simulink model "Controlador_PD"  (R2023a)
settings: Solver=ode1  StartTime=0.0  StopTime=10.0  FixedStep=0.01  RelTol=1e-3
settings Model: Creator=Nacho Andrade  LastModifiedBy=Nacho Andrade

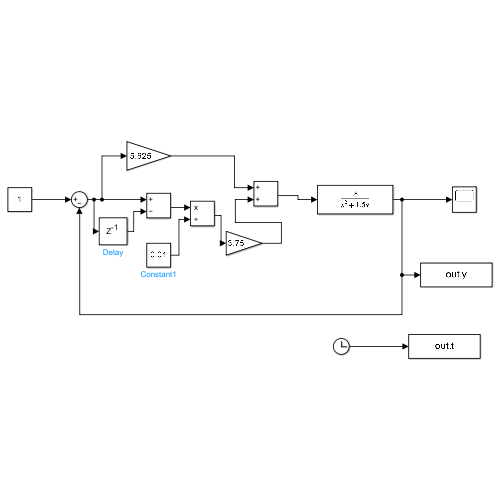
[thumbnail: Simulink's stored preview of the top-level diagram]
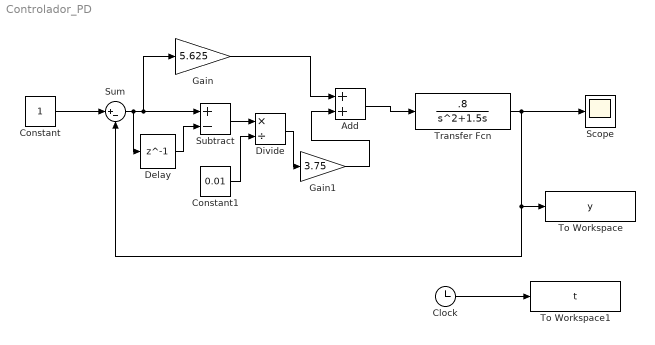
== system Controlador_PD ==
  Add : Sum
  Clock : Clock
  Constant : Constant
  Constant1 : Constant  Value=0.01
  Delay : Delay  DelayLength=1
  Divide : Product  Inputs=*/
  Gain : Gain  Gain=5.625
  Gain1 : Gain  Gain=3.75
  Scope : Scope
  Subtract : Sum  Inputs=+-
  Sum : Sum  Inputs=|+-
  To Workspace : ToWorkspace  VariableName=y  SampleTime=-1
  To Workspace1 : ToWorkspace  VariableName=t  SampleTime=-1
  Transfer Fcn : TransferFcn  Numerator=[.8]  Denominator=[1 1.5 0]
  wires:
  Constant/1 -> Sum/1
  Sum/1 -> Delay/1, Subtract/1, Gain/1
  Transfer Fcn/1 -> Sum/2, To Workspace/1, Scope/1
  Gain1/1 -> Add/2
  Add/1 -> Transfer Fcn/1
  Gain/1 -> Add/1
  Clock/1 -> To Workspace1/1
  Delay/1 -> Subtract/2
  Subtract/1 -> Divide/1
  Constant1/1 -> Divide/2
  Divide/1 -> Gain1/1
